simulink model "single_cmg_practice"  (R2023b)
settings: Solver=ode4  StartTime=0.0  StopTime=1000  FixedStep=0.001  RelTol=1e-3
undefined symbols (not defined in the file): As, Cube_L, F_vec, I_rw1, M_c, M_rw, sat, THR_Force, THR_Pos, torque_ext, X, Y, Z
libraries: sm_lib x391, nesl_utility x251, simulink_extras x103, sharedtransform x53, aerolibutil x30, sharedutil x13, simulink x12
(part 14 of 14)

== matlab function single_cmg_practice/Reaction_Wheel_Simple1/quaternion to Euler angle  ==
  data: angle output; q input
function angle = quat2eulang(q)
% ZYX 회전 가정

% q0 = q(1); q1 = q(2); q2 = q(3); q3 = q(4);
% 
% yaw = atan2(2*(q1*q2 + q0*q3), q0^2+q1^2-q2^2-q3^2);
% 
% s = 2*(q0*q2 - q3*q1);
% s = max(-1, min(1, s));      % clamp
% pitch = asin(s);
% 
% roll = atan2(2*(q2*q3 + q0*q1), q0^2-q1^2-q2^2+q3^2);



% % 'ZYX' 회전에서 DCM을 Body-frame -> 관성좌표계 으로 정의할 때, 각을 구하는 상황.
% % /                cos(psi) cos(theta),                              cos(theta) sin(psi),                   -sin(theta)     \
% % |                                                                                                                         |
% % | cos(psi) sin(phi) sin(theta) - cos(phi) sin(psi), cos(phi) cos(psi) + sin(phi) sin(psi) sin(theta), cos(theta) sin(phi) |
% % |                                                                                                                         |
% % \ sin(phi) sin(psi) + cos(phi) cos(psi) sin(theta), cos(phi) sin(psi) sin(theta) - cos(psi) sin(phi), cos(phi) cos(theta) /
R = quat2DCM(q);
yaw   = atan2(R(1,2), R(1,1));
pitch = -asin(R(1,3));
roll  = atan2(R(2,3), R(3,3));



% angle = [roll, pitch, yaw]';
angle = [yaw, pitch, roll]'; %MATLAB 에서는 [roll, pitch, yaw] 가 아닌 [yaw, pitch, roll] 순으로 값을 반환한다.
% 실제 도움말을 보면, 반환각 벡터에 대해 "Ψ is R1, Θ is R2, and Φ is R3." 으로 나와있는 것을 볼 수 있다.



function R = quat2DCM(q)

q0 = q(1); q1 = q(2); q2 = q(3); q3 = q(4);

%% DCM을 관성좌표계 -> Body-frame 으로 정의할 때의 행렬 
% R = [2*(q0^2 + q1^2)-1, 2*(q1*q2 - q0*q3),2*(q1*q3 + q2*q0);
%      2*(q1*q2 + q0*q3), 2*(q0^2 + q2^2)-1, 2*(q2*q3 - q1*q0);
%      2*(q1*q3 - q2*q0), 2*(q2*q3 + q1*q0), 2*(q0^2 + q3^2)-1];

%% DCM을 Body-frame -> 관성좌표계 으로 정의할 때의 행렬 
R = [q0^2+q1^2-q2^2-q3^2, 2*(q1*q2 + q0*q3), 2*(q1*q3 - q2*q0);
     2*(q1*q2 - q0*q3), q0^2-q1^2+q2^2-q3^2, 2*(q2*q3 + q1*q0);
     2*(q1*q3 + q2*q0), 2*(q2*q3 - q1*q0), q0^2-q1^2-q2^2+q3^2];

end

end

== matlab function single_cmg_practice/Prac1/rigid body ==
  data: t_ext input; omega_prime output; omega input
function omega_prime = fcn(t_ext, omega)
L = [0.3 0.3 0.3]'; %Length([m]) of cube 
M = 10; %Mass([kg]) of cube

% Density([kg/m^3]) of cube
density = M/(L(1)*L(2)*L(3));   
% MOI([kg*m^2]) of cube
I = [ 1/12*M*(L(2)^2+L(3)^2) 0 0;
      0 1/12*M*(L(1)^2+L(3)^2) 0;
      0 0 1/12*M*(L(1)^2+L(2)^2)];

omega_prime = inv(I)*(t_ext - cross(omega,I*omega));
